simulink model "air"  (R2016a)
settings: Solver=VariableStepAuto  StartTime=0.0  StopTime=10.0  RelTol=1e-3
settings Model: Creator=malikeh  LastModifiedBy=malikeh

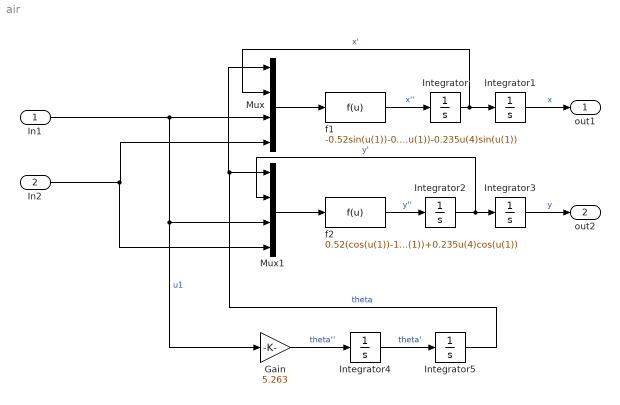
== system air ==
  In1 : Inport
  In2 : Inport  Port=2
  Gain : Gain  Gain=5.263
  Integrator{,1..5} (6 alike) : Integrator
  Mux : Mux
  Mux1 : Mux
  f1 : Fcn  Expr=-0.52sin(u(1))-0.0235u(2)+0.235u(3)cos(u(1))-0.235u(4)sin(u(1))
  f2 : Fcn  Expr=0.52(cos(u(1))-1)-0.0235u(2)+0.235u(3)sin(u(1))+0.235u(4)cos(u(1))
  out1 : Outport
  out2 : Outport  Port=2
  wires:
  f1/1 -> Integrator/1  "x''"
  f2/1 -> Integrator2/1  "y''"
  Integrator/1 -> Integrator1/1, Mux/2  "x'"
  Integrator2/1 -> Integrator3/1, Mux1/2  "y'"
  Mux/1 -> f1/1
  Mux1/1 -> f2/1
  Integrator4/1 -> Integrator5/1  "theta'"
  Gain/1 -> Integrator4/1  "theta''"
  Integrator5/1 -> Mux1/1, Mux/1  "theta"
  In1/1 -> Gain/1, Mux1/3, Mux/3  "u1"
  In2/1 -> Mux1/4, Mux/4
  Integrator1/1 -> out1/1  "x"
  Integrator3/1 -> out2/1  "y"
